simulink model "OilPLmp_DD"  (R2016b)
settings: configuration reference "CodeGenConfigSet" (kept outside this file)
values from neighbouring files (symbols this model uses):
  OILP_STOILPRESOPT_SY_C = Calibration.Parameter    [init_OilPLmp_DD.m]    (also in init_OilPLmp_DD_SIL.m = Simulink.Parameter)
  OilPLmp_aMin_C = Calibration.Parameter    [init_OilPLmp_DD.m]    (also in init_OilPLmp_DD_SIL.m = Simulink.Parameter)
  OilPLmp_nStrt1_C = Calibration.Parameter    [init_OilPLmp_DD.m]    (also in init_OilPLmp_DD_SIL.m = Simulink.Parameter)
  OilPLmp_nStrt2_C = Calibration.Parameter    [init_OilPLmp_DD.m]    (also in init_OilPLmp_DD_SIL.m = Simulink.Parameter)
  OilPLmp_stPsDiaDisbl_C = Calibration.Parameter    [init_OilPLmp_DD.m]    (also in init_OilPLmp_DD_SIL.m = Simulink.Parameter)
  OilPLmp_stPsDisbl_C = Calibration.Parameter    [init_OilPLmp_DD.m]    (also in init_OilPLmp_DD_SIL.m = Simulink.Parameter)
  OilPLmp_swtStrt_C = Calibration.Parameter    [init_OilPLmp_DD.m]    (also in init_OilPLmp_DD_SIL.m = Simulink.Parameter)
  OilPLmp_tiDebABSPos_C = Calibration.Parameter    [init_OilPLmp_DD.m]    (also in init_OilPLmp_DD_SIL.m = Simulink.Parameter)
  OilPLmp_tiInactv1_C = Calibration.Parameter    [init_OilPLmp_DD.m]    (also in init_OilPLmp_DD_SIL.m = Simulink.Parameter)
  OilPLmp_tiInactv2_C = Calibration.Parameter    [init_OilPLmp_DD.m]    (also in init_OilPLmp_DD_SIL.m = Simulink.Parameter)
  OilPLmp_tiStrt_C = Calibration.Parameter    [init_OilPLmp_DD.m]    (also in init_OilPLmp_DD_SIL.m = Simulink.Parameter)
  OilPLmp_vMin_C = Calibration.Parameter    [init_OilPLmp_DD.m]    (also in init_OilPLmp_DD_SIL.m = Simulink.Parameter)
undefined symbols (not defined in the file or in its folder): EngState_conv, OilPLmp_DD_DT
libraries: CXLib x5, simulink x2
settings Model: Creator=xinchangran  LastModifiedBy=xinchangran
settings ConfigSetRef: SourceLocation=Base Workspace

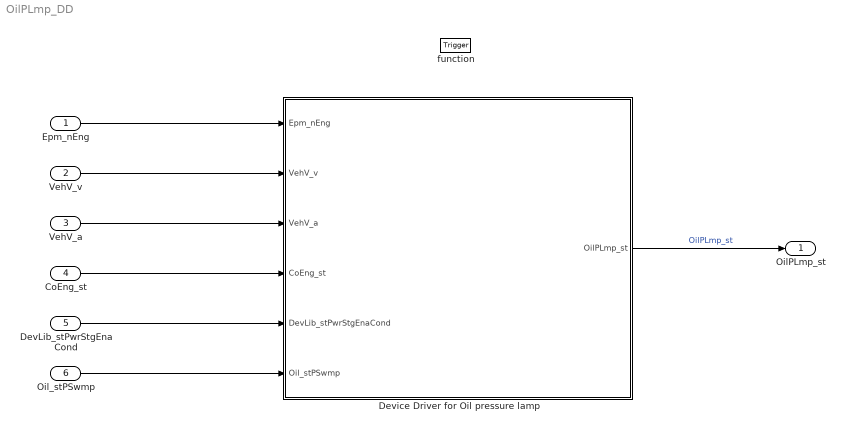
== system OilPLmp_DD ==
  Epm_nEng : Inport  Tag=rpm  Description=Engine speed  OutMin=0  OutMax=6000  OutDataTypeStr=EngSpeed_rpm
  VehV_v : Inport  Tag=km/h  Description=Vehicle speed  Port=2  OutMin=0  OutMax=250  OutDataTypeStr=VehSpeed_km_h
  VehV_a : Inport  Tag=m/s^2  Description=The acceleration of the vehicle  Port=3  OutMin=-32.7  OutMax=32.7  OutDataTypeStr=Acc_m_s2
  CoEng_st : Inport  Description=Engine coordinator state  Port=4  OutDataTypeStr=Enum: EngState_conv
  DevLib_stPwrStgEnaCond : Inport  Description=Control unit status relevant to power stage deactivation/error diagnosis  Port=5  OutMin=0  OutMax=65535  OutDataTypeStr=State_uint16
  Oil_stPSwmp : Inport  Description=sensor out oil pressure status  Port=6  OutMin=0  OutMax=1  OutDataTypeStr=boolean
  function : TriggerPort  TriggerType=function-call  VariantControl=Variant
  Device Driver for Oil pressure lamp : Subsystem
  OilPLmp_st : Outport  Description=oil pressure lamp status  OutMin=0  OutMax=1  OutDataTypeStr=boolean
  wires:
  Device Driver for Oil pressure lamp/1(OilPLmp_st) -> OilPLmp_st/1  "OilPLmp_st"
  CoEng_st/1 -> Device Driver for Oil pressure lamp/4(CoEng_st)
  VehV_a/1 -> Device Driver for Oil pressure lamp/3(VehV_a)
  VehV_v/1 -> Device Driver for Oil pressure lamp/2(VehV_v)
  Epm_nEng/1 -> Device Driver for Oil pressure lamp/1(Epm_nEng)
  DevLib_stPwrStgEnaCond/1 -> Device Driver for Oil pressure lamp/5(DevLib_stPwrStgEnaCond)
  Oil_stPSwmp/1 -> Device Driver for Oil pressure lamp/6(Oil_stPSwmp)

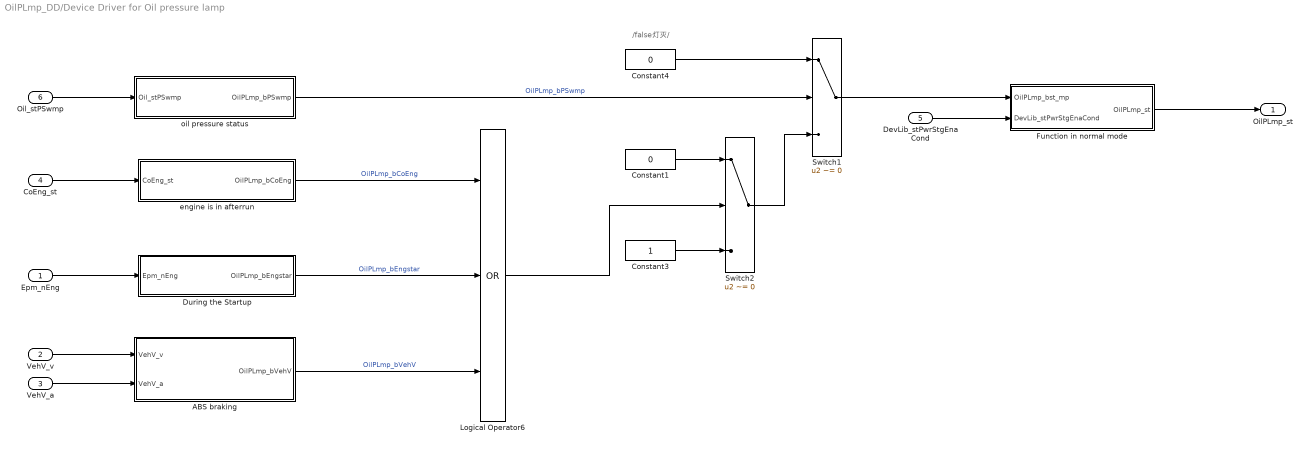
== system OilPLmp_DD/Device Driver for Oil pressure lamp ==
  note: /false灯灭/
  Epm_nEng : Inport
  VehV_v : Inport  Tag=km/h  Port=2
  VehV_a : Inport  Tag=m/s^2  Port=3
  CoEng_st : Inport  Port=4
  DevLib_stPwrStgEnaCond : Inport  Port=5
  Oil_stPSwmp : Inport  Port=6
  ABS braking : Subsystem
  Constant1 : Constant  Value=0  OutDataTypeStr=boolean
  Constant3 : Constant  OutDataTypeStr=boolean
  Constant4 : Constant  Value=0  OutDataTypeStr=boolean
  "During the Startup " : Subsystem
  Function in normal mode : Subsystem
  Logical Operator6 : Logic  Operator=OR  Inputs=3  AllPortsSameDT=off  OutDataTypeStr=boolean
  Switch1 : Switch  Criteria=u2 ~= 0  InputSameDT=on
  Switch2 : Switch  Criteria=u2 ~= 0  InputSameDT=on
  engine is in afterrun : Subsystem
  oil pressure status : Subsystem
  OilPLmp_st : Outport
  wires:
  "During the Startup "/1(OilPLmp_bEngstar) -> Logical Operator6/2  "OilPLmp_bEngstar"
  ABS braking/1(OilPLmp_bVehV) -> Logical Operator6/3  "OilPLmp_bVehV"
  engine is in afterrun/1(OilPLmp_bCoEng) -> Logical Operator6/1  "OilPLmp_bCoEng"
  oil pressure status/1(OilPLmp_bPSwmp) -> Switch1/2  "OilPLmp_bPSwmp"
  CoEng_st/1 -> engine is in afterrun/1(CoEng_st)
  VehV_v/1 -> ABS braking/1(VehV_v)
  VehV_a/1 -> ABS braking/2(VehV_a)
  Logical Operator6/1 -> Switch2/2
  DevLib_stPwrStgEnaCond/1 -> Function in normal mode/2(DevLib_stPwrStgEnaCond)
  Function in normal mode/1(OilPLmp_st) -> OilPLmp_st/1
  Oil_stPSwmp/1 -> oil pressure status/1(Oil_stPSwmp)
  Constant4/1 -> Switch1/1
  Switch1/1 -> Function in normal mode/1(OilPLmp_bst_mp)
  Switch2/1 -> Switch1/3
  Constant1/1 -> Switch2/1
  Constant3/1 -> Switch2/3
  Epm_nEng/1 -> "During the Startup "/1(Epm_nEng)

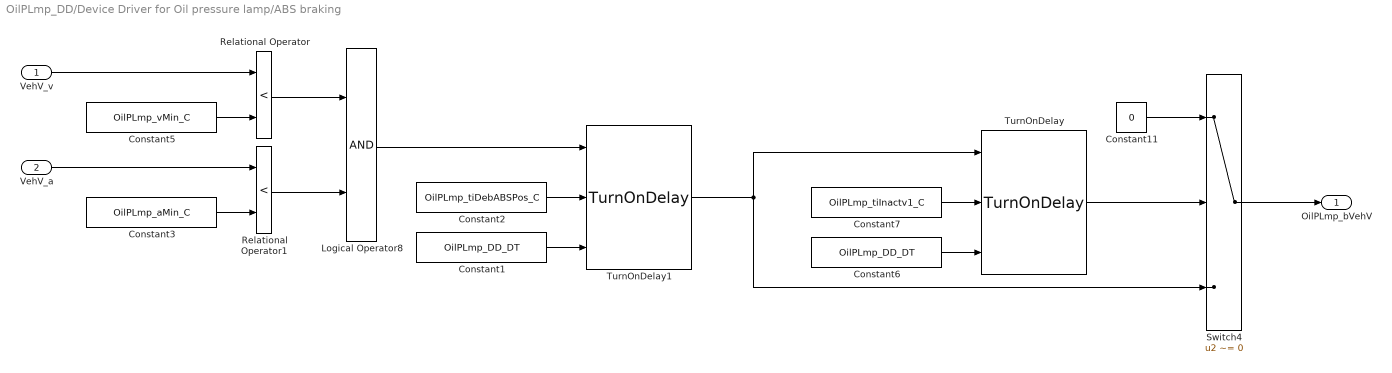
== system OilPLmp_DD/Device Driver for Oil pressure lamp/ABS braking ==
  VehV_v : Inport
  VehV_a : Inport  Port=2
  Constant1 : Constant  Value=OilPLmp_DD_DT
  Constant11 : Constant  Value=0  OutDataTypeStr=Inherit: Inherit via back propagation
  Constant2 : Constant  Value=OilPLmp_tiDebABSPos_C
  Constant3 : Constant  Value=OilPLmp_aMin_C
  Constant5 : Constant  Value=OilPLmp_vMin_C
  Constant6 : Constant  Value=OilPLmp_DD_DT
  Constant7 : Constant  Value=OilPLmp_tiInactv1_C
  Logical Operator8 : Logic  AllPortsSameDT=off  OutDataTypeStr=boolean
  Relational Operator : RelationalOperator  Operator=<  OutDataTypeStr=boolean  RndMeth=Simplest
  Relational Operator1 : RelationalOperator  Operator=<  OutDataTypeStr=boolean  RndMeth=Simplest
  Switch4 : Switch  Criteria=u2 ~= 0  InputSameDT=on
  TurnOnDelay : CXLib/TurnOnDelay
  TurnOnDelay1 : CXLib/TurnOnDelay
  OilPLmp_bVehV : Outport
  wires:
  Constant11/1 -> Switch4/1
  Switch4/1 -> OilPLmp_bVehV/1
  TurnOnDelay1/1 -> TurnOnDelay/1, Switch4/3
  Constant5/1 -> Relational Operator/2
  VehV_v/1 -> Relational Operator/1
  Relational Operator/1 -> Logical Operator8/1
  Constant3/1 -> Relational Operator1/2
  VehV_a/1 -> Relational Operator1/1
  Relational Operator1/1 -> Logical Operator8/2
  Constant7/1 -> TurnOnDelay/2
  Constant6/1 -> TurnOnDelay/3
  TurnOnDelay/1 -> Switch4/2
  Logical Operator8/1 -> TurnOnDelay1/1
  Constant2/1 -> TurnOnDelay1/2
  Constant1/1 -> TurnOnDelay1/3

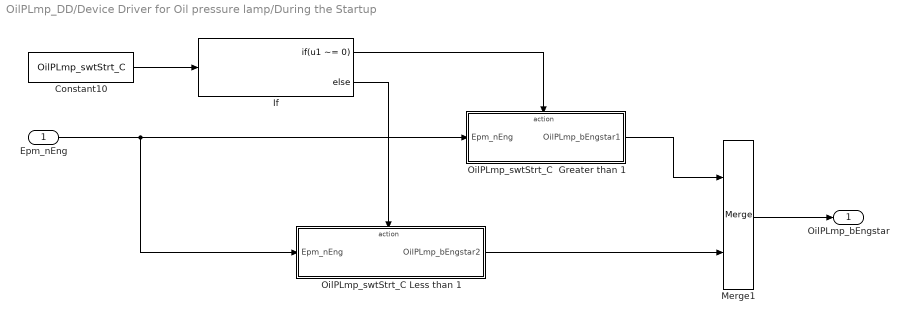
== system OilPLmp_DD/Device Driver for Oil pressure lamp/During the Startup  ==
  Epm_nEng : Inport
  Constant10 : Constant  Value=OilPLmp_swtStrt_C
  If : If  IfExpression=u1 ~= 0
  Merge1 : Merge
  OilPLmp_swtStrt_C  Greater than 1 : Subsystem  TreatAsAtomicUnit=on
  OilPLmp_swtStrt_C Less than 1 : Subsystem  TreatAsAtomicUnit=on
  OilPLmp_bEngstar : Outport
  wires:
  Merge1/1 -> OilPLmp_bEngstar/1
  OilPLmp_swtStrt_C  Greater than 1/1(OilPLmp_bEngstar1) -> Merge1/1
  OilPLmp_swtStrt_C Less than 1/1(OilPLmp_bEngstar2) -> Merge1/2
  Epm_nEng/1 -> OilPLmp_swtStrt_C Less than 1/1(Epm_nEng), OilPLmp_swtStrt_C  Greater than 1/1(Epm_nEng)
  Constant10/1 -> If/1
  If/1 -> OilPLmp_swtStrt_C  Greater than 1/Action
  If/2 -> OilPLmp_swtStrt_C Less than 1/Action

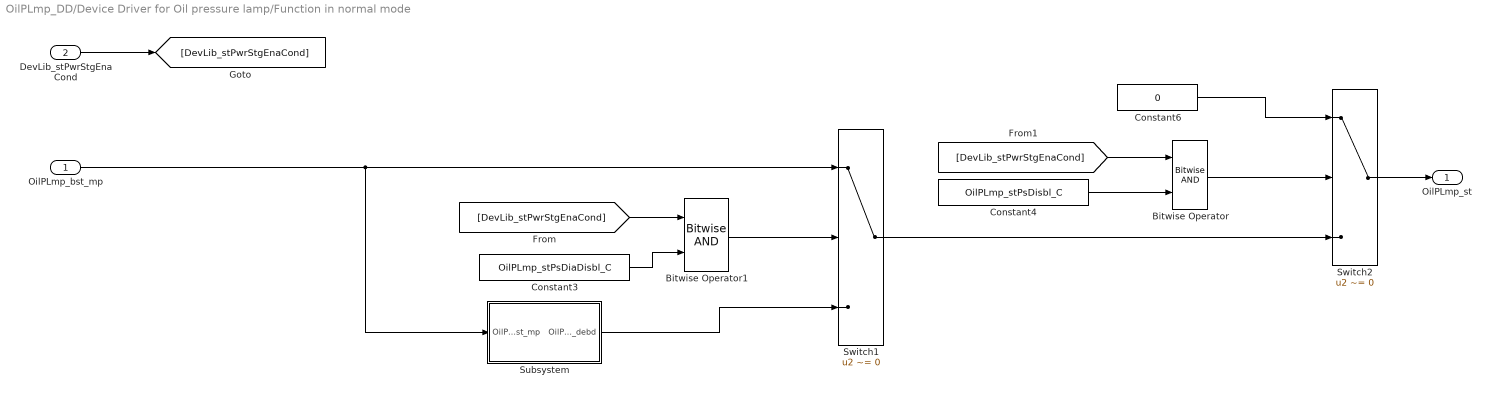
== system OilPLmp_DD/Device Driver for Oil pressure lamp/Function in normal mode ==
  OilPLmp_bst_mp : Inport
  DevLib_stPwrStgEnaCond : Inport  Port=2
  Bitwise Operator : simulink/Logic and Bit Operations/Bitwise Operator  logicop=AND  UseBitMask=off  NumInputPorts=2  BitMask=bin2dec('11011001')  BitMaskRealWorld=Stored Integer
  Bitwise Operator1 : simulink/Logic and Bit Operations/Bitwise Operator  logicop=AND  UseBitMask=off  NumInputPorts=2  BitMask=bin2dec('11011001')  BitMaskRealWorld=Stored Integer
  Constant3 : Constant  Value=OilPLmp_stPsDiaDisbl_C  SampleTime=-1
  Constant4 : Constant  Value=OilPLmp_stPsDisbl_C  SampleTime=-1
  Constant6 : Constant  Value=0  OutDataTypeStr=Inherit: Inherit via back propagation  SampleTime=-1
  Subsystem : Subsystem
      mask Display: disp('Error Handing')
  Switch1 : Switch  Criteria=u2 ~= 0  InputSameDT=on
  Switch2 : Switch  Criteria=u2 ~= 0  InputSameDT=on
  OilPLmp_st : Outport
  wires:
  Constant6/1 -> Switch2/1
  Switch1/1 -> Switch2/3
  Subsystem/1(OilPLmp_bst_debd) -> Switch1/3
  Switch2/1 -> OilPLmp_st/1
  Bitwise Operator/1 -> Switch2/2
  OilPLmp_bst_mp/1 -> Subsystem/1(OilPLmp_bst_mp), Switch1/1
  Bitwise Operator1/1 -> Switch1/2
  DevLib_stPwrStgEnaCond/1 -> [DevLib_stPwrStgEnaCond]
  [DevLib_stPwrStgEnaCond] -> Bitwise Operator/1
  Constant4/1 -> Bitwise Operator/2
  [DevLib_stPwrStgEnaCond] -> Bitwise Operator1/1
  Constant3/1 -> Bitwise Operator1/2

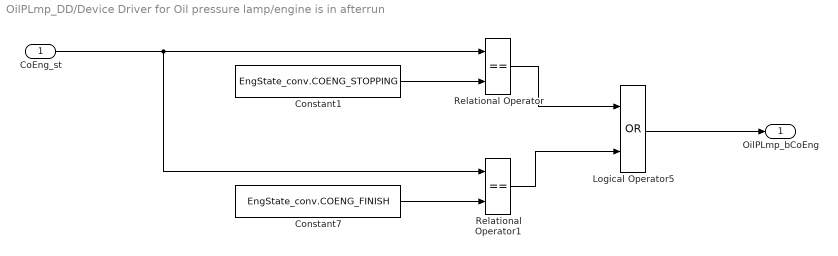
== system OilPLmp_DD/Device Driver for Oil pressure lamp/engine is in afterrun ==
  CoEng_st : Inport
  Constant1 : Constant  Value=EngState_conv.COENG_STOPPING
  Constant7 : Constant  Value=EngState_conv.COENG_FINISH
  Logical Operator5 : Logic  Operator=OR  AllPortsSameDT=off  OutDataTypeStr=boolean
  Relational Operator : RelationalOperator  Operator===  OutDataTypeStr=boolean  RndMeth=Simplest
  Relational Operator1 : RelationalOperator  Operator===  OutDataTypeStr=boolean  RndMeth=Simplest
  OilPLmp_bCoEng : Outport
  wires:
  Logical Operator5/1 -> OilPLmp_bCoEng/1
  CoEng_st/1 -> Relational Operator1/1, Relational Operator/1
  Constant1/1 -> Relational Operator/2
  Constant7/1 -> Relational Operator1/2
  Relational Operator/1 -> Logical Operator5/1
  Relational Operator1/1 -> Logical Operator5/2

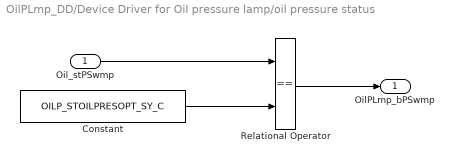
== system OilPLmp_DD/Device Driver for Oil pressure lamp/oil pressure status ==
  Oil_stPSwmp : Inport
  Constant : Constant  Value=OILP_STOILPRESOPT_SY_C
  Relational Operator : RelationalOperator  Operator===  OutDataTypeStr=boolean  RndMeth=Simplest
  OilPLmp_bPSwmp : Outport
  wires:
  Relational Operator/1 -> OilPLmp_bPSwmp/1
  Oil_stPSwmp/1 -> Relational Operator/1
  Constant/1 -> Relational Operator/2

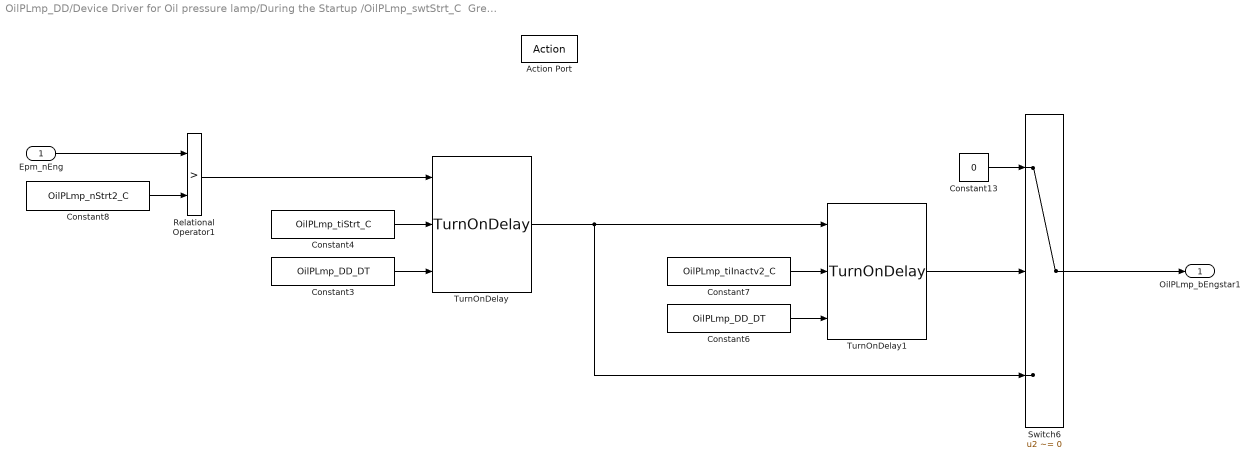
== system OilPLmp_DD/Device Driver for Oil pressure lamp/During the Startup /OilPLmp_swtStrt_C  Greater than 1 ==
  Epm_nEng : Inport
  Action Port : ActionPort  ActionType=then
  Constant13 : Constant  Value=0  OutDataTypeStr=Inherit: Inherit via back propagation
  Constant3 : Constant  Value=OilPLmp_DD_DT
  Constant4 : Constant  Value=OilPLmp_tiStrt_C
  Constant6 : Constant  Value=OilPLmp_DD_DT
  Constant7 : Constant  Value=OilPLmp_tiInactv2_C
  Constant8 : Constant  Value=OilPLmp_nStrt2_C
  Relational Operator1 : RelationalOperator  Operator=>  OutDataTypeStr=boolean  RndMeth=Simplest
  Switch6 : Switch  Criteria=u2 ~= 0  InputSameDT=on
  TurnOnDelay : CXLib/TurnOnDelay
  TurnOnDelay1 : CXLib/TurnOnDelay
  OilPLmp_bEngstar1 : Outport
  wires:
  Relational Operator1/1 -> TurnOnDelay/1
  Constant7/1 -> TurnOnDelay1/2
  Constant6/1 -> TurnOnDelay1/3
  Constant13/1 -> Switch6/1
  Constant3/1 -> TurnOnDelay/3
  TurnOnDelay/1 -> TurnOnDelay1/1, Switch6/3
  Switch6/1 -> OilPLmp_bEngstar1/1
  Constant8/1 -> Relational Operator1/2
  TurnOnDelay1/1 -> Switch6/2
  Constant4/1 -> TurnOnDelay/2
  Epm_nEng/1 -> Relational Operator1/1

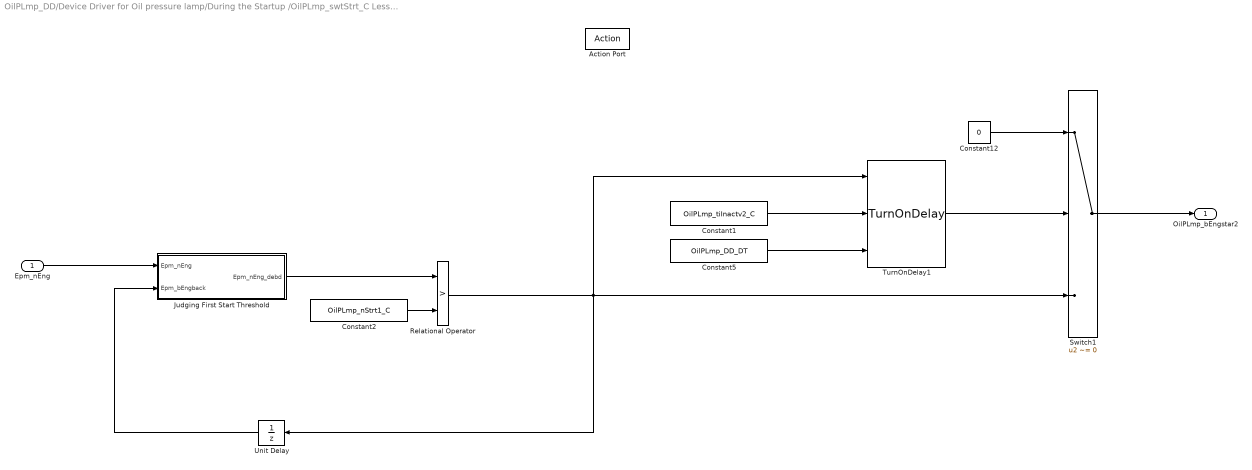
== system OilPLmp_DD/Device Driver for Oil pressure lamp/During the Startup /OilPLmp_swtStrt_C Less than 1 ==
  Epm_nEng : Inport
  Action Port : ActionPort  ActionType=else
  Constant1 : Constant  Value=OilPLmp_tiInactv2_C
  Constant12 : Constant  Value=0  OutDataTypeStr=Inherit: Inherit via back propagation
  Constant2 : Constant  Value=OilPLmp_nStrt1_C
  Constant5 : Constant  Value=OilPLmp_DD_DT
  Judging First Start Threshold : Subsystem
  Relational Operator : RelationalOperator  Operator=>  OutDataTypeStr=boolean  RndMeth=Simplest
  Switch1 : Switch  Criteria=u2 ~= 0  InputSameDT=on
  TurnOnDelay1 : CXLib/TurnOnDelay
  Unit Delay : UnitDelay  SampleTime=-1
      settings: AttributesFormatString=InitialValue=%<InitialCondition>
  OilPLmp_bEngstar2 : Outport
  wires:
  Judging First Start Threshold/1(Epm_nEng_debd) -> Relational Operator/1
  Unit Delay/1 -> Judging First Start Threshold/2(Epm_bEngback)
  Constant1/1 -> TurnOnDelay1/2
  Constant2/1 -> Relational Operator/2
  Relational Operator/1 -> TurnOnDelay1/1, Switch1/3, Unit Delay/1
  Constant12/1 -> Switch1/1
  Constant5/1 -> TurnOnDelay1/3
  Switch1/1 -> OilPLmp_bEngstar2/1
  TurnOnDelay1/1 -> Switch1/2
  Epm_nEng/1 -> Judging First Start Threshold/1(Epm_nEng)

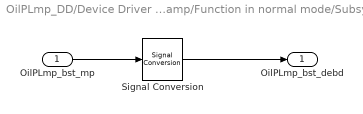
== system OilPLmp_DD/Device Driver for Oil pressure lamp/Function in normal mode/Subsystem ==
  OilPLmp_bst_mp : Inport
  Signal Conversion : SignalConversion  OverrideOpt=off
  OilPLmp_bst_debd : Outport
  wires:
  OilPLmp_bst_mp/1 -> Signal Conversion/1
  Signal Conversion/1 -> OilPLmp_bst_debd/1

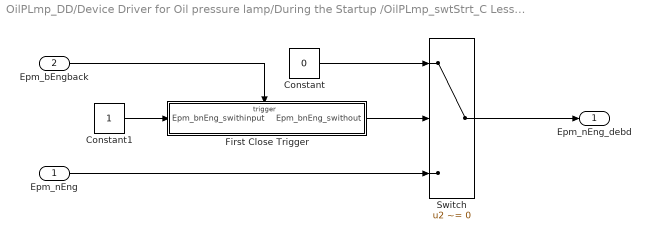
== system OilPLmp_DD/Device Driver for Oil pressure lamp/During the Startup /OilPLmp_swtStrt_C Less than 1/Judging First Start Threshold ==
  Epm_nEng : Inport
  Epm_bEngback : Inport  Port=2
  Constant : Constant  Value=0  OutDataTypeStr=Inherit: Inherit via back propagation
  Constant1 : Constant  OutDataTypeStr=boolean
  "First Close Trigger " : Subsystem  TreatAsAtomicUnit=on
  Switch : Switch  Criteria=u2 ~= 0  InputSameDT=on
  Epm_nEng_debd : Outport
  wires:
  Switch/1 -> Epm_nEng_debd/1
  Epm_bEngback/1 -> "First Close Trigger "/Trigger
  Epm_nEng/1 -> Switch/3
  "First Close Trigger "/1(Epm_bnEng_swithout) -> Switch/2
  Constant/1 -> Switch/1
  Constant1/1 -> "First Close Trigger "/1(Epm_bnEng_swithinput)

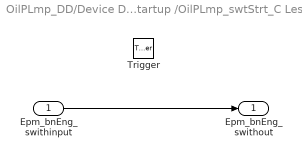
== system OilPLmp_DD/Device Driver for Oil pressure lamp/During the Startup /OilPLmp_swtStrt_C Less than 1/Judging First Start Threshold/First Close Trigger  ==
  Epm_bnEng_swithinput : Inport
  Trigger : TriggerPort  TriggerType=falling  VariantControl=Variant
  Epm_bnEng_swithout : Outport
  wires:
  Epm_bnEng_swithinput/1 -> Epm_bnEng_swithout/1
